simulink model "electric_drives_control"  (R2019a)
settings: Solver=ode45  StartTime=0.0  StopTime=8  MaxStep=1e-5  RelTol=1e-3
libraries: powerlib x4, simulink x1
settings Model: Creator=shaosimin  LastModifiedBy=shaosimin

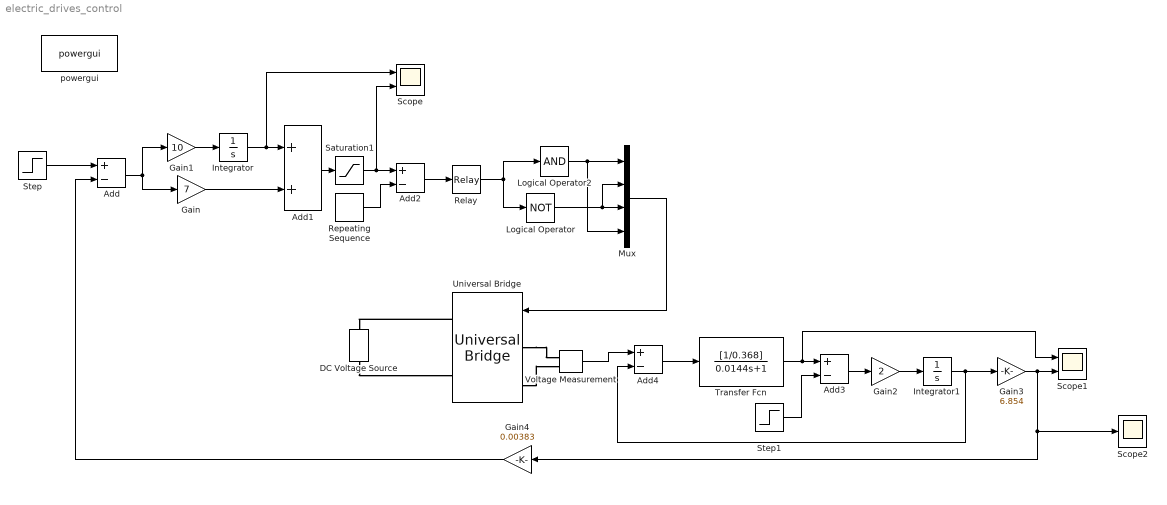
== system electric_drives_control ==
  Add{,2..4} (4 alike) : Sum  Inputs=+-
  Add1 : Sum
  DC Voltage Source : powerlib/Electrical Sources/DC Voltage Source  Amplitude=538  Measurements=None
      settings: SourceProductName=Simscape Electrical
  Gain : Gain  Gain=7
  Gain1 : Gain  Gain=10
  Gain2 : Gain  Gain=2
  Gain3 : Gain  Gain=6.854
  Gain4 : Gain  Gain=0.00383
  Integrator : Integrator  LimitOutput=on  UpperSaturationLimit=5  LowerSaturationLimit=-5
  Integrator1 : Integrator  UpperSaturationLimit=5  LowerSaturationLimit=-5
  Logical Operator : Logic  Operator=NOT  AllPortsSameDT=off
  Logical Operator2 : Logic  Inputs=1  AllPortsSameDT=off
  Mux : Mux
  Relay : Relay
  Repeating Sequence : simulink/Sources/Repeating Sequence  rep_seq_t=[0 0.125e-3]  rep_seq_y=[-5 5]
  Saturation1 : Saturate  UpperLimit=4.998  LowerLimit=-4.998
  Scope : Scope  NumInputPorts=2
  Scope1 : Scope  NumInputPorts=2
  Scope2 : Scope
  Step : Step  Time=0  After=10  SampleTime=0
  Step1 : Step  Time=0  SampleTime=0
  Transfer Fcn : TransferFcn  Numerator=[1/0.368]  Denominator=[0.0144 1]
  Universal Bridge : powerlib/Power Electronics/Universal Bridge  Arms=2  SnubberResistance=1e5  SnubberCapacitance=inf  Device=MOSFET / Diodes  Ron=1e-3  Lon=0  ForwardVoltages="[  0  0  ]"  ForwardVoltage=0  GTOparameters=[ 10e-6 , 20e-6 ]  IGBTparameters=[ 1e-6 , 2e-6 ]  Measurements=Device voltages  Measurements_2=None  converterType=Rectifier
      settings: SourceProductName=Simscape Electrical
  Voltage Measurement : powerlib/Measurements/Voltage Measurement  PhasorSimulation=off  OutputType=Complex  PSBequivalent=0
      settings: SourceProductName=Simscape Electrical
  powergui : powerlib/powergui  Priority=1  SimulationMode=Continuous  SampleTime=50e-6  frequency=60  Iterations=50  frequencyindice=0  Pbase=100e6  ErrMax=1e-4  UnitsV=kV  UnitsW=MW  buscounter=0  FunctionMessages=off  echomessages=off  EnableUseOfTLC=off  CurrentSourceSwitches=off  DisableSnubberDevices=off  DisableRonSwitches=off  DisableVfSwitches=off  DisplayEquations=off  AutomaticDiscreteSolvers=off  SolverType=Tustin/Backward Euler (TBE)  Interpol=off  ExternalGateDelay=off  methode=off  Ts=100  x0status=blocks  SPID=on  SwTol=0  HookPort=off  NonlinearTolerance=0  nMaxIteration=15  ContinueOnMaxIteration=off  RestoreLinks=warning  ResistiveCurrentMeasurement=off  Frange=[0:2:500]  Ylog=off  Xlog=on  ShowGrid=off  save=off  variable=ZData  structure=0  ZoomFFT=off  StartTime=0.0  cycles=1  DisplayStyle=1  fundamental=60  FreqAxis=off  MaxFrequency=1000  frequencyindicesteady=1  RmsSteady=1  display=off
      settings: SourceProductName=Simscape Electrical
  wires:
  Step/1 -> Add/1
  Add/1 -> Gain/1, Gain1/1
  Gain1/1 -> Integrator/1
  Integrator/1 -> Scope/1, Add1/1
  Gain/1 -> Add1/2
  Add1/1 -> Saturation1/1
  Saturation1/1 -> Scope/2, Add2/1
  Repeating Sequence/1 -> Add2/2
  Add2/1 -> Relay/1
  Relay/1 -> Logical Operator2/1, Logical Operator/1
  Logical Operator/1 -> Mux/2, Mux/3
  Mux/1 -> Universal Bridge/1
  Transfer Fcn/1 -> Scope1/1, Add3/1
  Step1/1 -> Add3/2
  Add3/1 -> Gain2/1
  Gain2/1 -> Integrator1/1
  Integrator1/1 -> Gain3/1, Add4/2
  Gain3/1 -> Scope2/1, Gain4/1, Scope1/2
  Gain4/1 -> Add/2
  Logical Operator2/1 -> Mux/1, Mux/4
  Add4/1 -> Transfer Fcn/1
  Voltage Measurement/1 -> Add4/1
  connections:
  Universal Bridge/RConn1 -- DC Voltage Source/RConn1
  DC Voltage Source/LConn1 -- Universal Bridge/RConn2
  Universal Bridge/LConn1 -- Voltage Measurement/LConn1
  Universal Bridge/LConn2 -- Voltage Measurement/LConn2
